simulink model "Simulation"  (R2019a)
settings: Solver=ode2  StartTime=0.0  StopTime=30  FixedStep=0.01  RelTol=1e-3
settings Model: Creator=DELL  LastModifiedBy=DELL
settings SolverCC: AlgebraicLoopSolver=LineSearch

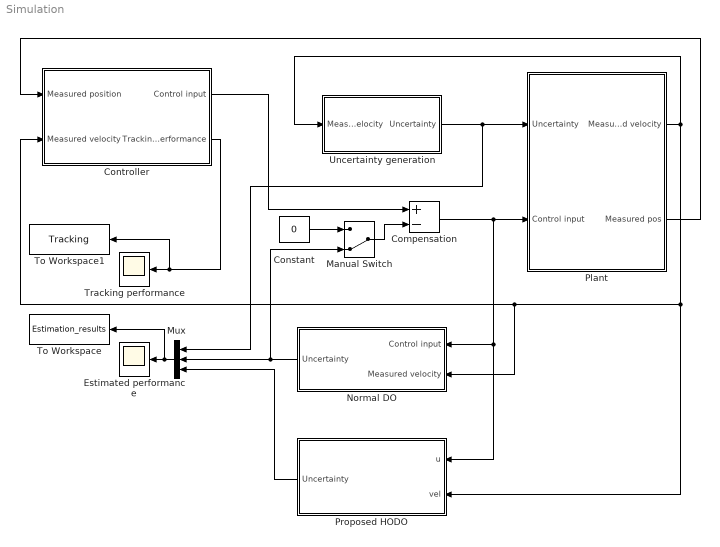
== system Simulation ==
  Compensation : Sum  Inputs=+-
  Constant : Constant  Value=0
  Controller : Subsystem
  Estimated performance : Scope
  Manual Switch : ManualSwitch  CurrentSetting=0
  Mux : Mux  Inputs=3
  Normal DO : Subsystem
  Plant : Subsystem
  Proposed HODO : Subsystem
  To Workspace : ToWorkspace  VariableName=Estimation_results  SaveFormat=Structure With Time  SampleTime=-1
  To Workspace1 : ToWorkspace  VariableName=Tracking  SaveFormat=Structure With Time  SampleTime=-1
  Tracking performance : Scope
  Uncertainty generation : Subsystem  TreatAsAtomicUnit=on
  wires:
  Uncertainty generation/1(Uncertainty) -> Mux/1, Plant/1(Uncertainty)
  Controller/1(Control input) -> Compensation/1
  Normal DO/1(Uncertainty) -> Manual Switch/2, Mux/2
  Constant/1 -> Manual Switch/1
  Manual Switch/1 -> Compensation/2
  Mux/1 -> To Workspace/1, Estimated performance/1
  Plant/2(Measured pos) -> Controller/1(Measured position)
  Plant/1(Measured velocity) -> Normal DO/2(Measured velocity), Controller/2(Measured velocity), Proposed HODO/2(vel), Uncertainty generation/1(Measured velocity)
  Compensation/1 -> Plant/2(Control input), Proposed HODO/1(u), Normal DO/1(Control input)
  Proposed HODO/1(Uncertainty) -> Mux/3
  Controller/2(Tracking performance) -> To Workspace1/1, Tracking performance/1

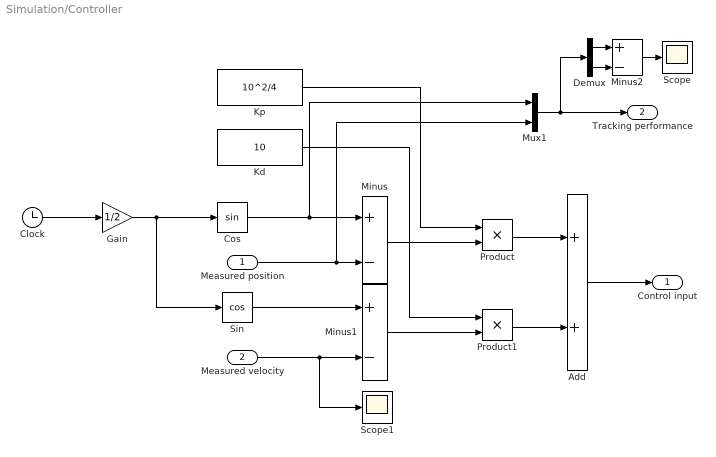
== system Simulation/Controller ==
  Measured position : Inport
  Measured velocity : Inport  Port=2
  Add : Sum
  Clock : Clock
  Cos : Trigonometry
  Demux : Demux  Outputs=2
  Gain : Gain  Gain=1/2
  Kd : Constant  Value=10
  Kp : Constant  Value=10^2/4
  Minus : Sum  Inputs=+-
  Minus1 : Sum  Inputs=+-
  Minus2 : Sum  Inputs=+-
  Mux1 : Mux  Inputs=2
  Product : Product
  Product1 : Product
  Scope : Scope
  Scope1 : Scope
  Sin : Trigonometry  Operator=cos
  Control input : Outport
  Tracking performance : Outport  Port=2
  wires:
  Minus/1 -> Product/2
  Measured velocity/1 -> Scope1/1, Minus1/2
  Minus1/1 -> Product1/2
  Product/1 -> Add/1
  Measured position/1 -> Mux1/2, Minus/2
  Product1/1 -> Add/2
  Add/1 -> Control input/1
  Cos/1 -> Mux1/1, Minus/1
  Kp/1 -> Product/1
  Kd/1 -> Product1/1
  Mux1/1 -> Tracking performance/1, Demux/1
  Demux/1 -> Minus2/1
  Demux/2 -> Minus2/2
  Minus2/1 -> Scope/1
  Clock/1 -> Gain/1
  Sin/1 -> Minus1/1
  Gain/1 -> Cos/1, Sin/1

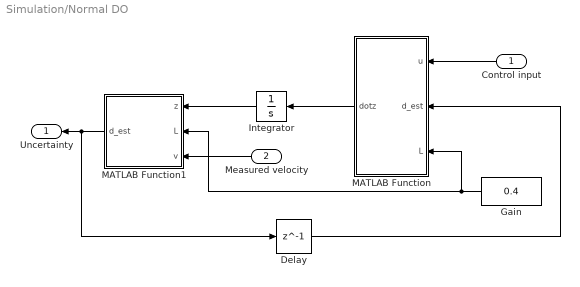
== system Simulation/Normal DO ==
  Control input : Inport
  Measured velocity : Inport  Port=2
  Delay : Delay  DelayLength=1
  Gain : Constant  Value=0.4
  Integrator : Integrator
  MATLAB Function : MATLAB Function  TreatAsAtomicUnit=on
  MATLAB Function1 : MATLAB Function  TreatAsAtomicUnit=on
  Uncertainty : Outport
  wires:
  Measured velocity/1 -> MATLAB Function1/3(v)
  Gain/1 -> MATLAB Function/3(L), MATLAB Function1/2(L)
  Integrator/1 -> MATLAB Function1/1(z)
  Delay/1 -> MATLAB Function/2(d_est)
  MATLAB Function1/1(d_est) -> Delay/1, Uncertainty/1
  MATLAB Function/1(dotz) -> Integrator/1
  Control input/1 -> MATLAB Function/1(u)

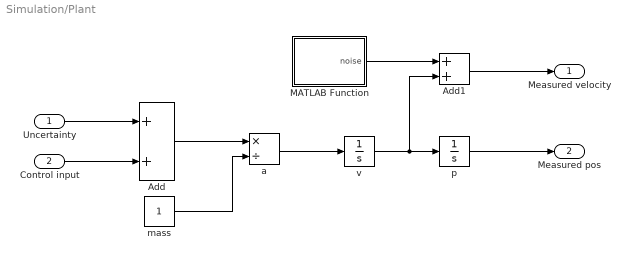
== system Simulation/Plant ==
  Uncertainty : Inport
  Control input : Inport  Port=2
  Add : Sum
  Add1 : Sum
  MATLAB Function : MATLAB Function  TreatAsAtomicUnit=on
  a : Product  Inputs=*/
  mass : Constant
  p : Integrator
  v : Integrator
  Measured velocity : Outport
  Measured pos : Outport  Port=2
  wires:
  v/1 -> Add1/2, p/1
  mass/1 -> a/2
  Control input/1 -> Add/2
  p/1 -> Measured pos/1
  Add/1 -> a/1
  Uncertainty/1 -> Add/1
  Add1/1 -> Measured velocity/1
  MATLAB Function/1(noise) -> Add1/1
  a/1 -> v/1

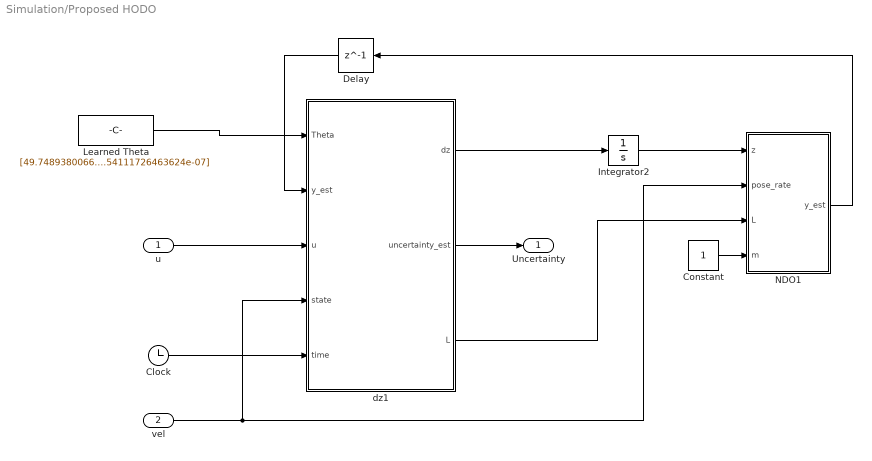
== system Simulation/Proposed HODO ==
  u : Inport
  vel : Inport  Port=2
  Clock : Clock
  Constant : Constant
  Delay : Delay  DelayLength=1
  Integrator2 : Integrator
  Learned Theta : Constant  Value="[49.7489380066717\t2.15538475056842e-06\t-0.499991140946822\t-9.99956635104724\t-8.81248048534289e-07\t-3.61775579804657e-06\t0.249981529109538\t3.772170061336976e-08\t1.54111726463624e-07]"
  NDO1 : MATLAB Function  TreatAsAtomicUnit=on
  dz1 : MATLAB Function  TreatAsAtomicUnit=on
  Uncertainty : Outport
  wires:
  NDO1/1(y_est) -> Delay/1
  Delay/1 -> dz1/2(y_est)
  dz1/3(L) -> NDO1/3(L)
  dz1/2(uncertainty_est) -> Uncertainty/1
  u/1 -> dz1/3(u)
  Clock/1 -> dz1/5(time)
  dz1/1(dz) -> Integrator2/1
  Integrator2/1 -> NDO1/1(z)
  vel/1 -> NDO1/2(pose_rate), dz1/4(state)
  Constant/1 -> NDO1/4(m)
  Learned Theta/1 -> dz1/1(Theta)

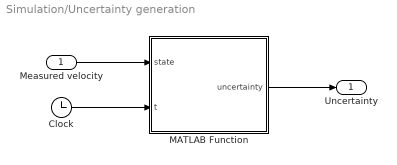
== system Simulation/Uncertainty generation ==
  Measured velocity : Inport
  Clock : Clock
  MATLAB Function : MATLAB Function  TreatAsAtomicUnit=on
  Uncertainty : Outport
  wires:
  Clock/1 -> MATLAB Function/2(t)
  MATLAB Function/1(uncertainty) -> Uncertainty/1
  Measured velocity/1 -> MATLAB Function/1(state)

== matlab function Simulation/Plant/MATLAB Function ==
  data: noise output
function noise = fcn()

 %% Noise generation
var_noise = 0.1; 
noise = wgn(1, 1, 10*log10(var_noise));

== matlab function Simulation/Normal DO/MATLAB Function ==
  data: u input; dotz output; d_est input; L input
function dotz = fcn(u,d_est,L)
dotz = -L*(u + d_est);

== matlab function Simulation/Normal DO/MATLAB Function1 ==
  data: z input size=1; d_est output; L input size=1; v input size=1
function d_est  = fcn(z, L, v)
m = 1;
d_est = z + L*v.*m;

== matlab function Simulation/Uncertainty generation/MATLAB Function ==
  data: state input; uncertainty output; t input
function uncertainty = fcn(state, t)


%% Uncertainty 

% uncertainty = sin(t)* sin(state) + 2;
% uncertainty = state - 1/12 * state^3 -1/4*t^2 ;
% uncertainty = -1/9 * sin(state)* t^3;

uncertainty = [-state^2 + 50, -10, 0.5] * [1, t, t^2]';

== matlab function Simulation/Proposed HODO/NDO1 ==
  data: z input size=3; y_est output size=3; pose_rate input; L input; m input
function y_est = fcn(z,pose_rate,L, m)

p = L .* m .* pose_rate(1);

y_est = z + p;

== matlab function Simulation/Proposed HODO/dz1 ==
  data: Theta input size=[1, 9]; y_est input size=3; dz output size=3; u input; state input; uncertainty_est output; L output; time input
function [dz, uncertainty_est, L] = fcn(Theta,y_est,u, state, time)

%% Initial parameters
p = 2;
A = zeros(p+1, p+1);
for i = 2:1:(p+1)
    A(i, i-1) = i-1;
end
D = zeros(p+1, p+1);
D(1,1) = 1;
D(2,2) = 1;
for i = 3:1:p+1
    D_shift = zeros(1, p+1);
    D_shift(1, 2:p+1) = D(i-1, 1:p);
    D(i, :) = 2.* D_shift - D(i-2,:);
end

%% Output matrix of uncertainty system
C = Theta * B_X_fun(state, p) * D;

%% The design of observer gain
%% K. Chen and A. Astolfi, “Adaptive control for systems with time-varying parameters,” 
%% IEEE Transactions on Automatic Control, vol. 66, no. 5, pp. 1986–2001.
M = [C; C * A; C * A * A];
rank_M = rank(M);
inv_M =  inv(M);

theta = 1;
Delta_theta = diag([1/theta, 1/theta^2, 1/theta^3]);
inv_Delta_theta = diag([theta, theta^2, theta^3]);

A_k = [0 1 0; 0 0 1; 0 0 0];
C_k = [1 0 0];
P1 = [0 0 1; 0 1 0; 1 0 0];
P_k = P1 * [C_k; C_k * A_k; C_k * A_k * A_k];
% L_k = [8 12 6]';          %% pole -2
L_k = [0.16*0.4 0.48 1.2]'; %% pole -0.4
K = pinv(P_k) * L_k;

L = inv(M) * inv_Delta_theta * K;
gain = A - L * C; 
[~, eee] = eig(gain);
eigval = diag(eee);

%% Observer
dz = A * y_est - L*(u + C * y_est);
uncertainty_est = C * y_est;

%% Test the accuracy of Theta
uncertainty_2 = Theta * B_X_fun(state, p) * xi_fun(time, p);
end

function B_X = B_X_fun(x, p)
 n = length(x);
 m = 1;   % The matched disturbance
 s1 = (p+1)^(m+n);
 s2 = (p+1)^(m);
 PI = zeros((p+1)^(n), 1);
 B_X = zeros(s1, s2);
 
 for i = 1:1:(p+1)^(n)
     k_str     = dec2base(i-1,(p+1));
     k_length  = length(k_str);
     PI(i,1) = 1;
     for j = 1:1:k_length
      PI(i,1) =  PI(i,1)*Cheby_poly(single(str2double(k_str(k_length+1-j))), x(j));
     end
 end
 
 for j = 1:1:s2
    B_X(:, j) = [zeros(1, (j-1)*(p+1)^n) PI' zeros(1, s1-j*(p+1)^n)];
 end
end

function xi = xi_fun(time_stamp, p)
 m = 1;
 s2 = (p+1)^(m);
 xi = zeros(s2, 1);
 
 for i = 1:1:s2
      xi(i,1) =  Cheby_poly(i-1, time_stamp);
 end
end
 

function poly = Cheby_poly(order, var)
  if order == 0
    poly = 1;
  elseif order == 1
    poly = var;
%   elseif order == 2
%     poly = 2 * var^2 - 1;
%   elseif order == 3
%     poly = 4 * var^3 - 3 * var;
%    elseif order == 10
%     poly = 512*var^10 - 1280*var^8 + 1120*var^6 -400 *var*4 + 50 *var^2 -1;
  else
    poly = 2*var*Cheby_poly(order-1, var)- Cheby_poly(order-2, var);
  end
end
